simulink model "RRR_Robot_Control"  (R2021a)
settings: Solver=FixedStepAuto  StartTime=0.0  StopTime=10.0  FixedStep=0.001  RelTol=1e-3
values from neighbouring files (symbols this model uses):
  a = M\b    [parameters_Values.m]
  g = 9.81    [parameters_Values.m]
  L = [0.1,0.4,0.3]    [parameters_Values.m]
  m = [0.1,0.3,0.2]    [parameters_Values.m]
  r1 = 0.025    [parameters_Values.m]
libraries: pid_lib x3
settings Model: Creator=power  LastModifiedBy=power

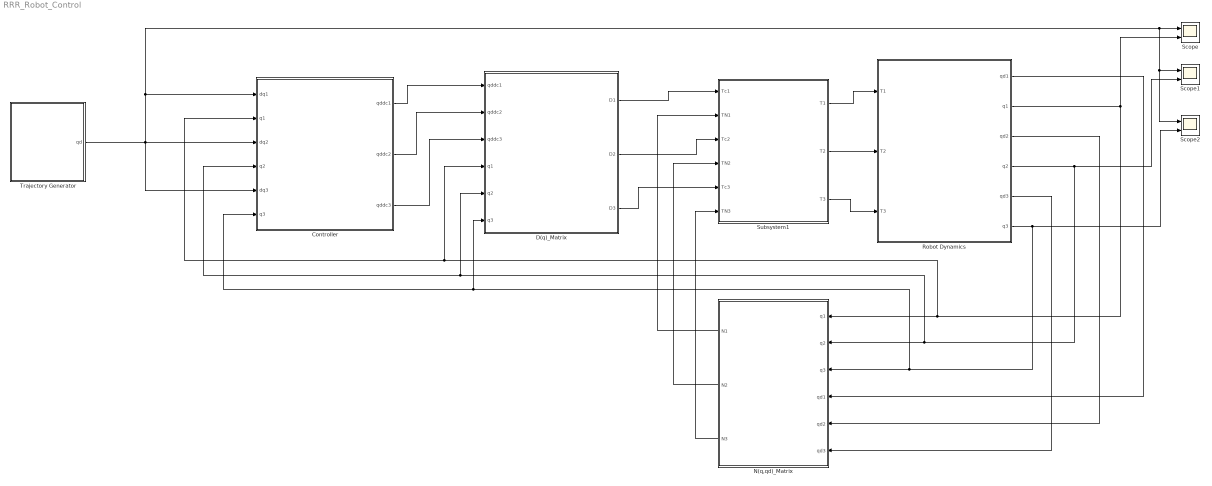
== system RRR_Robot_Control ==
  Controller : Subsystem
  D(q)_Matrix : Subsystem
  N(q,qd)_Matrix : Subsystem
  Robot Dynamics : Subsystem
  Scope : Scope  NumInputPorts=2
  Scope1 : Scope  NumInputPorts=2
  Scope2 : Scope  NumInputPorts=2
  Subsystem1 : Subsystem
  Trajectory Generator : Subsystem
  wires:
  Subsystem1/2(T2) -> Robot Dynamics/2(T2)
  Subsystem1/1(T1) -> Robot Dynamics/1(T1)
  Subsystem1/3(T3) -> Robot Dynamics/3(T3)
  N(q,qd)_Matrix/1(N1) -> Subsystem1/2(TN1)
  N(q,qd)_Matrix/2(N2) -> Subsystem1/4(TN2)
  N(q,qd)_Matrix/3(N3) -> Subsystem1/6(TN3)
  D(q)_Matrix/1(D1) -> Subsystem1/1(Tc1)
  D(q)_Matrix/2(D2) -> Subsystem1/3(Tc2)
  D(q)_Matrix/3(D3) -> Subsystem1/5(Tc3)
  Robot Dynamics/2(q1) -> Scope/2, Controller/2(q1), D(q)_Matrix/4(q1), N(q,qd)_Matrix/1(q1)
  Robot Dynamics/6(q3) -> Scope2/2, Controller/6(q3), D(q)_Matrix/6(q3), N(q,qd)_Matrix/3(q3)
  Robot Dynamics/4(q2) -> Scope1/2, Controller/4(q2), D(q)_Matrix/5(q2), N(q,qd)_Matrix/2(q2)
  Robot Dynamics/1(qd1) -> N(q,qd)_Matrix/4(qd1)
  Robot Dynamics/3(qd2) -> N(q,qd)_Matrix/5(qd2)
  Robot Dynamics/5(qd3) -> N(q,qd)_Matrix/6(qd3)
  Controller/1(qddc1) -> D(q)_Matrix/1(qddc1)
  Controller/2(qddc2) -> D(q)_Matrix/2(qddc2)
  Controller/3(qddc3) -> D(q)_Matrix/3(qddc3)
  Trajectory Generator/1(qd) -> Controller/5(dq3), Controller/3(dq2), Scope2/1, Scope1/1, Scope/1, Controller/1(dq1)

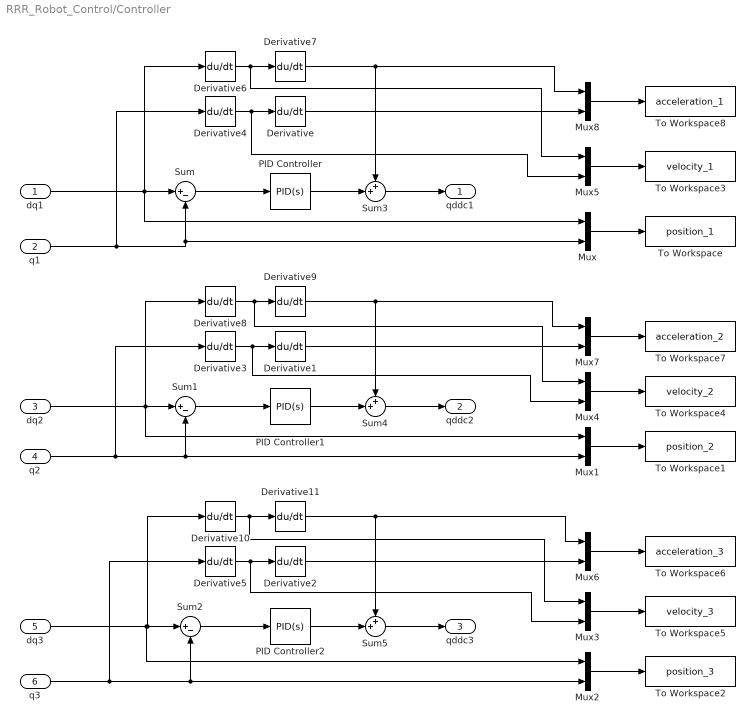
== system RRR_Robot_Control/Controller ==
  dq1 : Inport
  q1 : Inport  Port=2
  dq2 : Inport  Port=3
  q2 : Inport  Port=4
  dq3 : Inport  Port=5
  q3 : Inport  Port=6
  Derivative{,1..11} (12 alike) : Derivative
  Mux{,1..8} (9 alike) : Mux  Inputs=2
  PID Controller : pid_lib/PID Controller  Controller=PID  Form=Parallel  TimeDomain=Continuous-time  UseExternalTs=off  SampleTime=-1  IntegratorMethod=Forward Euler  FilterMethod=Forward Euler  ControllerParametersSource=internal  P=1  I=1  D=1  UseFilter=on  N=100  TunerSelectOption=Transfer Function Based (PID Tuner App)  InitialConditionSource=internal  InitialConditionForIntegrator=0  InitialConditionForFilter=0  DifferentiatorICPrevScaledInput=0  ExternalReset=none  TrackingMode=off  Kt=1  LimitOutput=off  SatLimitsSource=internal  UpperSaturationLimit=inf  LowerSaturationLimit=-inf  LinearizeAsGain=on  AntiWindupMode=none  Kb=1  POutMin=[]  POutMax=[]  IOutMin=[]  IOutMax=[]  DOutMin=[]  DOutMax=[]  NOutMin=[]  NOutMax=[]  SumOutMin=[]  SumOutMax=[]  SaturationOutMin=[]  SaturationOutMax=[]  PParamMin=[]  PParamMax=[]  IParamMin=[]  IParamMax=[]  DParamMin=[]  DParamMax=[]  NParamMin=[]  NParamMax=[]  KbParamMin=[]  KbParamMax=[]  KtParamMin=[]  KtParamMax=[]  KbOutMin=[]  KbOutMax=[]  KtOutMin=[]  KtOutMax=[]  IntegratorOutMin=[]  IntegratorOutMax=[]  FilterOutMin=[]  FilterOutMax=[]  SumI1OutMin=[]  SumI1OutMax=[]  SumI2OutMin=[]  SumI2OutMax=[]  SumI3OutMin=[]  SumI3OutMax=[]  SumI4OutMin=[]  SumI4OutMax=[]  SumDOutMin=[]  SumDOutMax=[]  DifferentiatorOutMin=[]  DifferentiatorOutMax=[]  FilterDiffOutCoefMin=[]  FilterDiffOutCoefMax=[]  ReciprocalOutMin=[]  ReciprocalOutMax=[]  SumDenOutMin=[]  SumDenOutMax=[]  SumNumOutMin=[]  SumNumOutMax=[]  DivideOutMin=[]  DivideOutMax=[]  UdiffTsProdOutMin=[]  UdiffTsProdOutMax=[]  NTsProdOutMin=[]  NTsProdOutMax=[]  UintegralTsProdOutMin=[]  UintegralTsProdOutMax=[]  UngainTsProdOutMin=[]  UngainTsProdOutMax=[]  IntegratorContinuousStateAttributes=''  IntegratorStateMustResolveToSignalObject=off  IntegratorRTWStateStorageClass=Auto  FilterContinuousStateAttributes=''  FilterStateMustResolveToSignalObject=off  FilterRTWStateStorageClass=Auto  ParallelPVariant=InternalParameters  IdealPVariant=Disabled  IVariant=InternalParameters  DVariant=InternalParameters  IntegratorVariant=Continuous  SatVariant=Disabled  AWVariant=Passthrough  PCopyVariant=Disabled  TRVariant=Disabled  FdbkBlocksVariant=Forward  IdealPFdbkVariant=Disabled  SatFdbkVariant=Disabled  DerivativeFilterVariant=ContFilter  NVariant=InternalParameters  NCopyVariant=Disabled  FilterICVariant=InternalICsFilter  IntegratorICVariant=InternalICs  ExternalResetVariant=Disabled  TRSumVariant=Passthrough  SumFdbkVariant=Disabled  SumVariant=Sum_PID  TsampFilterVariant=InternalTs  TsampNgainVariant=Passthrough  TsampIntegralVariant=Passthrough  ExternalSaturationOutDataTypeStr=Inherit: Same as second input
  PID Controller1 : pid_lib/PID Controller  Controller=PID  Form=Parallel  TimeDomain=Continuous-time  UseExternalTs=off  SampleTime=-1  IntegratorMethod=Forward Euler  FilterMethod=Forward Euler  ControllerParametersSource=internal  P=1  I=1  D=1  UseFilter=on  N=100  TunerSelectOption=Transfer Function Based (PID Tuner App)  InitialConditionSource=internal  InitialConditionForIntegrator=0  InitialConditionForFilter=0  DifferentiatorICPrevScaledInput=0  ExternalReset=none  TrackingMode=off  Kt=1  LimitOutput=off  SatLimitsSource=internal  UpperSaturationLimit=inf  LowerSaturationLimit=-inf  LinearizeAsGain=on  AntiWindupMode=none  Kb=1  POutMin=[]  POutMax=[]  IOutMin=[]  IOutMax=[]  DOutMin=[]  DOutMax=[]  NOutMin=[]  NOutMax=[]  SumOutMin=[]  SumOutMax=[]  SaturationOutMin=[]  SaturationOutMax=[]  PParamMin=[]  PParamMax=[]  IParamMin=[]  IParamMax=[]  DParamMin=[]  DParamMax=[]  NParamMin=[]  NParamMax=[]  KbParamMin=[]  KbParamMax=[]  KtParamMin=[]  KtParamMax=[]  KbOutMin=[]  KbOutMax=[]  KtOutMin=[]  KtOutMax=[]  IntegratorOutMin=[]  IntegratorOutMax=[]  FilterOutMin=[]  FilterOutMax=[]  SumI1OutMin=[]  SumI1OutMax=[]  SumI2OutMin=[]  SumI2OutMax=[]  SumI3OutMin=[]  SumI3OutMax=[]  SumI4OutMin=[]  SumI4OutMax=[]  SumDOutMin=[]  SumDOutMax=[]  DifferentiatorOutMin=[]  DifferentiatorOutMax=[]  FilterDiffOutCoefMin=[]  FilterDiffOutCoefMax=[]  ReciprocalOutMin=[]  ReciprocalOutMax=[]  SumDenOutMin=[]  SumDenOutMax=[]  SumNumOutMin=[]  SumNumOutMax=[]  DivideOutMin=[]  DivideOutMax=[]  UdiffTsProdOutMin=[]  UdiffTsProdOutMax=[]  NTsProdOutMin=[]  NTsProdOutMax=[]  UintegralTsProdOutMin=[]  UintegralTsProdOutMax=[]  UngainTsProdOutMin=[]  UngainTsProdOutMax=[]  IntegratorContinuousStateAttributes=''  IntegratorStateMustResolveToSignalObject=off  IntegratorRTWStateStorageClass=Auto  FilterContinuousStateAttributes=''  FilterStateMustResolveToSignalObject=off  FilterRTWStateStorageClass=Auto  ParallelPVariant=InternalParameters  IdealPVariant=Disabled  IVariant=InternalParameters  DVariant=InternalParameters  IntegratorVariant=Continuous  SatVariant=Disabled  AWVariant=Passthrough  PCopyVariant=Disabled  TRVariant=Disabled  FdbkBlocksVariant=Forward  IdealPFdbkVariant=Disabled  SatFdbkVariant=Disabled  DerivativeFilterVariant=ContFilter  NVariant=InternalParameters  NCopyVariant=Disabled  FilterICVariant=InternalICsFilter  IntegratorICVariant=InternalICs  ExternalResetVariant=Disabled  TRSumVariant=Passthrough  SumFdbkVariant=Disabled  SumVariant=Sum_PID  TsampFilterVariant=InternalTs  TsampNgainVariant=Passthrough  TsampIntegralVariant=Passthrough  ExternalSaturationOutDataTypeStr=Inherit: Same as second input
  PID Controller2 : pid_lib/PID Controller  Controller=PID  Form=Parallel  TimeDomain=Continuous-time  UseExternalTs=off  SampleTime=-1  IntegratorMethod=Forward Euler  FilterMethod=Forward Euler  ControllerParametersSource=internal  P=1  I=1  D=1  UseFilter=on  N=100  TunerSelectOption=Transfer Function Based (PID Tuner App)  InitialConditionSource=internal  InitialConditionForIntegrator=0  InitialConditionForFilter=0  DifferentiatorICPrevScaledInput=0  ExternalReset=none  TrackingMode=off  Kt=1  LimitOutput=off  SatLimitsSource=internal  UpperSaturationLimit=inf  LowerSaturationLimit=-inf  LinearizeAsGain=on  AntiWindupMode=none  Kb=1  POutMin=[]  POutMax=[]  IOutMin=[]  IOutMax=[]  DOutMin=[]  DOutMax=[]  NOutMin=[]  NOutMax=[]  SumOutMin=[]  SumOutMax=[]  SaturationOutMin=[]  SaturationOutMax=[]  PParamMin=[]  PParamMax=[]  IParamMin=[]  IParamMax=[]  DParamMin=[]  DParamMax=[]  NParamMin=[]  NParamMax=[]  KbParamMin=[]  KbParamMax=[]  KtParamMin=[]  KtParamMax=[]  KbOutMin=[]  KbOutMax=[]  KtOutMin=[]  KtOutMax=[]  IntegratorOutMin=[]  IntegratorOutMax=[]  FilterOutMin=[]  FilterOutMax=[]  SumI1OutMin=[]  SumI1OutMax=[]  SumI2OutMin=[]  SumI2OutMax=[]  SumI3OutMin=[]  SumI3OutMax=[]  SumI4OutMin=[]  SumI4OutMax=[]  SumDOutMin=[]  SumDOutMax=[]  DifferentiatorOutMin=[]  DifferentiatorOutMax=[]  FilterDiffOutCoefMin=[]  FilterDiffOutCoefMax=[]  ReciprocalOutMin=[]  ReciprocalOutMax=[]  SumDenOutMin=[]  SumDenOutMax=[]  SumNumOutMin=[]  SumNumOutMax=[]  DivideOutMin=[]  DivideOutMax=[]  UdiffTsProdOutMin=[]  UdiffTsProdOutMax=[]  NTsProdOutMin=[]  NTsProdOutMax=[]  UintegralTsProdOutMin=[]  UintegralTsProdOutMax=[]  UngainTsProdOutMin=[]  UngainTsProdOutMax=[]  IntegratorContinuousStateAttributes=''  IntegratorStateMustResolveToSignalObject=off  IntegratorRTWStateStorageClass=Auto  FilterContinuousStateAttributes=''  FilterStateMustResolveToSignalObject=off  FilterRTWStateStorageClass=Auto  ParallelPVariant=InternalParameters  IdealPVariant=Disabled  IVariant=InternalParameters  DVariant=InternalParameters  IntegratorVariant=Continuous  SatVariant=Disabled  AWVariant=Passthrough  PCopyVariant=Disabled  TRVariant=Disabled  FdbkBlocksVariant=Forward  IdealPFdbkVariant=Disabled  SatFdbkVariant=Disabled  DerivativeFilterVariant=ContFilter  NVariant=InternalParameters  NCopyVariant=Disabled  FilterICVariant=InternalICsFilter  IntegratorICVariant=InternalICs  ExternalResetVariant=Disabled  TRSumVariant=Passthrough  SumFdbkVariant=Disabled  SumVariant=Sum_PID  TsampFilterVariant=InternalTs  TsampNgainVariant=Passthrough  TsampIntegralVariant=Passthrough  ExternalSaturationOutDataTypeStr=Inherit: Same as second input
  Sum : Sum  Inputs=|+-
  Sum1 : Sum  Inputs=|+-
  Sum2 : Sum  Inputs=|+-
  Sum3 : Sum  Inputs=++|
  Sum4 : Sum  Inputs=++|
  Sum5 : Sum  Inputs=++|
  To Workspace : ToWorkspace  VariableName=position_1  SaveFormat=Timeseries  SampleTime=0.05
  To Workspace1 : ToWorkspace  VariableName=position_2  SaveFormat=Timeseries  SampleTime=0.05
  To Workspace2 : ToWorkspace  VariableName=position_3  SaveFormat=Timeseries  SampleTime=0.05
  To Workspace3 : ToWorkspace  VariableName=velocity_1  SaveFormat=Timeseries  SampleTime=0.05
  To Workspace4 : ToWorkspace  VariableName=velocity_2  SaveFormat=Timeseries  SampleTime=0.05
  To Workspace5 : ToWorkspace  VariableName=velocity_3  SaveFormat=Timeseries  SampleTime=0.05
  To Workspace6 : ToWorkspace  VariableName=acceleration_3  SaveFormat=Timeseries  SampleTime=0.05
  To Workspace7 : ToWorkspace  VariableName=acceleration_2  SaveFormat=Timeseries  SampleTime=0.05
  To Workspace8 : ToWorkspace  VariableName=acceleration_1  SaveFormat=Timeseries  SampleTime=0.05
  qddc1 : Outport
  qddc2 : Outport  Port=2
  qddc3 : Outport  Port=3
  wires:
  Sum/1 -> PID Controller/1
  Sum1/1 -> PID Controller1/1
  Sum2/1 -> PID Controller2/1
  dq1/1 -> Derivative6/1, Mux/1, Sum/1
  q1/1 -> Derivative4/1, Sum/2, Mux/2
  dq2/1 -> Derivative8/1, Mux1/1, Sum1/1
  q2/1 -> Derivative3/1, Mux1/2, Sum1/2
  dq3/1 -> Mux2/1, Derivative10/1, Sum2/1
  q3/1 -> Derivative5/1, Sum2/2, Mux2/2
  PID Controller2/1 -> Sum5/2
  Sum5/1 -> qddc3/1
  Derivative2/1 -> Mux6/2
  Sum4/1 -> qddc2/1
  PID Controller1/1 -> Sum4/2
  Sum3/1 -> qddc1/1
  PID Controller/1 -> Sum3/2
  Derivative3/1 -> Mux4/2, Derivative1/1
  Derivative4/1 -> Mux5/2, Derivative/1
  Derivative5/1 -> Mux3/2, Derivative2/1
  Derivative/1 -> Mux8/2
  Derivative1/1 -> Mux7/2
  Mux/1 -> To Workspace/1
  Mux1/1 -> To Workspace1/1
  Mux2/1 -> To Workspace2/1
  Mux3/1 -> To Workspace5/1
  Mux4/1 -> To Workspace4/1
  Mux5/1 -> To Workspace3/1
  Derivative6/1 -> Mux5/1, Derivative7/1
  Derivative8/1 -> Mux4/1, Derivative9/1
  Derivative10/1 -> Mux3/1, Derivative11/1
  Mux6/1 -> To Workspace6/1
  Derivative11/1 -> Sum5/1, Mux6/1
  Mux7/1 -> To Workspace7/1
  Derivative9/1 -> Sum4/1, Mux7/1
  Mux8/1 -> To Workspace8/1
  Derivative7/1 -> Sum3/1, Mux8/1

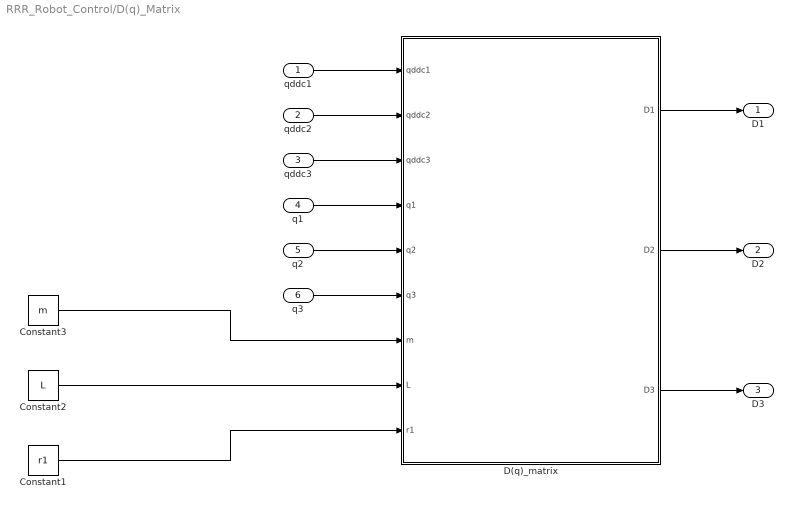
== system RRR_Robot_Control/D(q)_Matrix ==
  qddc1 : Inport
  qddc2 : Inport  Port=2
  qddc3 : Inport  Port=3
  q1 : Inport  Port=4
  q2 : Inport  Port=5
  q3 : Inport  Port=6
  Constant1 : Constant  Value=r1
  Constant2 : Constant  Value=L
  Constant3 : Constant  Value=m
  D(q)_matrix : MATLAB Function  TreatAsAtomicUnit=on
  D1 : Outport
  D2 : Outport  Port=2
  D3 : Outport  Port=3
  wires:
  D(q)_matrix/1(D1) -> D1/1
  D(q)_matrix/2(D2) -> D2/1
  D(q)_matrix/3(D3) -> D3/1
  qddc1/1 -> D(q)_matrix/1(qddc1)
  qddc2/1 -> D(q)_matrix/2(qddc2)
  qddc3/1 -> D(q)_matrix/3(qddc3)
  Constant1/1 -> D(q)_matrix/9(r1)
  Constant2/1 -> D(q)_matrix/8(L)
  Constant3/1 -> D(q)_matrix/7(m)
  q1/1 -> D(q)_matrix/4(q1)
  q2/1 -> D(q)_matrix/5(q2)
  q3/1 -> D(q)_matrix/6(q3)

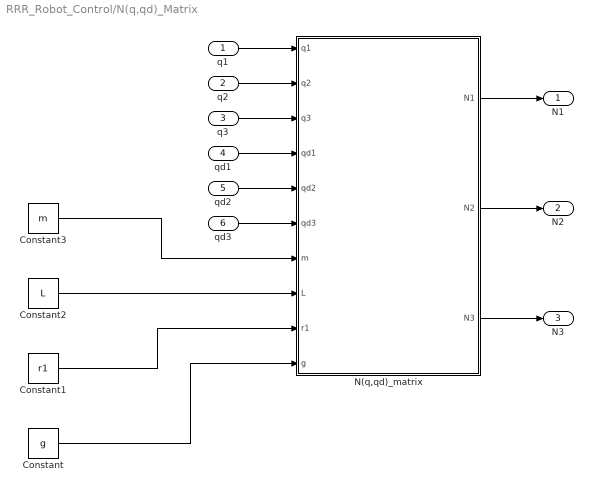
== system RRR_Robot_Control/N(q,qd)_Matrix ==
  q1 : Inport
  q2 : Inport  Port=2
  q3 : Inport  Port=3
  qd1 : Inport  Port=4
  qd2 : Inport  Port=5
  qd3 : Inport  Port=6
  Constant : Constant  Value=g
  Constant1 : Constant  Value=r1
  Constant2 : Constant  Value=L
  Constant3 : Constant  Value=m
  N(q,qd)_matrix : MATLAB Function  TreatAsAtomicUnit=on
  N1 : Outport
  N2 : Outport  Port=2
  N3 : Outport  Port=3
  wires:
  q1/1 -> N(q,qd)_matrix/1(q1)
  N(q,qd)_matrix/1(N1) -> N1/1
  N(q,qd)_matrix/2(N2) -> N2/1
  N(q,qd)_matrix/3(N3) -> N3/1
  q2/1 -> N(q,qd)_matrix/2(q2)
  q3/1 -> N(q,qd)_matrix/3(q3)
  qd2/1 -> N(q,qd)_matrix/5(qd2)
  qd1/1 -> N(q,qd)_matrix/4(qd1)
  qd3/1 -> N(q,qd)_matrix/6(qd3)
  Constant/1 -> N(q,qd)_matrix/10(g)
  Constant1/1 -> N(q,qd)_matrix/9(r1)
  Constant2/1 -> N(q,qd)_matrix/8(L)
  Constant3/1 -> N(q,qd)_matrix/7(m)

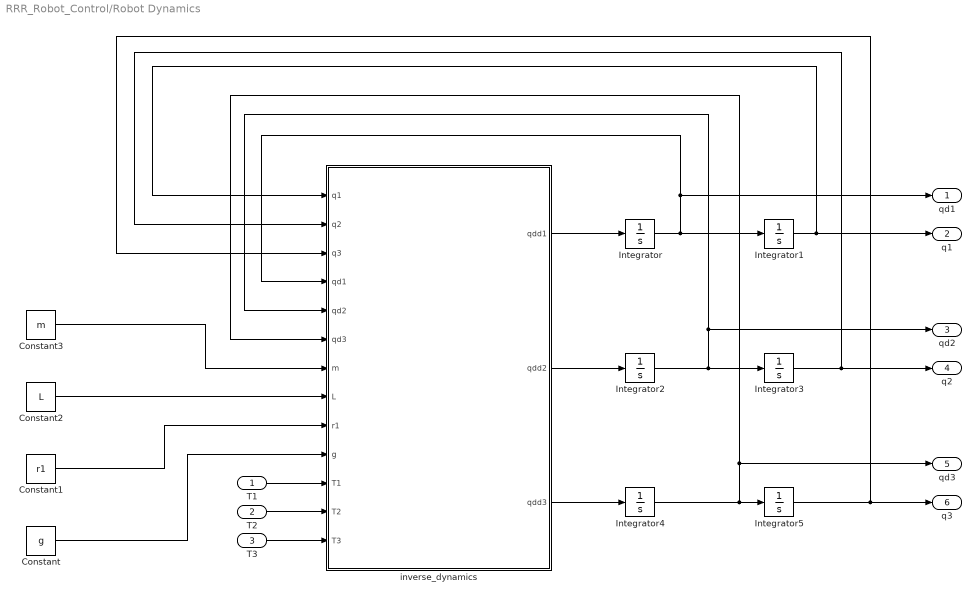
== system RRR_Robot_Control/Robot Dynamics ==
  T1 : Inport
  T2 : Inport  Port=2
  T3 : Inport  Port=3
  Constant : Constant  Value=g
  Constant1 : Constant  Value=r1
  Constant2 : Constant  Value=L
  Constant3 : Constant  Value=m
  Integrator{,1..5} (6 alike) : Integrator
  inverse_dynamics : MATLAB Function  TreatAsAtomicUnit=on
  qd1 : Outport
  q1 : Outport  Port=2
  qd2 : Outport  Port=3
  q2 : Outport  Port=4
  qd3 : Outport  Port=5
  q3 : Outport  Port=6
  wires:
  T1/1 -> inverse_dynamics/11(T1)
  inverse_dynamics/1(qdd1) -> Integrator/1
  Integrator/1 -> qd1/1, inverse_dynamics/4(qd1), Integrator1/1
  Integrator1/1 -> q1/1, inverse_dynamics/1(q1)
  inverse_dynamics/2(qdd2) -> Integrator2/1
  Integrator2/1 -> qd2/1, inverse_dynamics/5(qd2), Integrator3/1
  inverse_dynamics/3(qdd3) -> Integrator4/1
  Integrator4/1 -> qd3/1, inverse_dynamics/6(qd3), Integrator5/1
  Integrator5/1 -> q3/1, inverse_dynamics/3(q3)
  Constant/1 -> inverse_dynamics/10(g)
  Constant1/1 -> inverse_dynamics/9(r1)
  Constant2/1 -> inverse_dynamics/8(L)
  Constant3/1 -> inverse_dynamics/7(m)
  Integrator3/1 -> inverse_dynamics/2(q2), q2/1
  T2/1 -> inverse_dynamics/12(T2)
  T3/1 -> inverse_dynamics/13(T3)

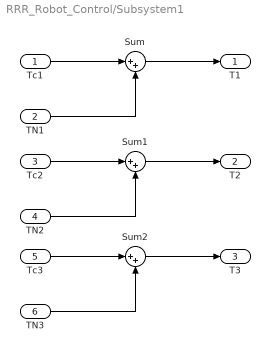
== system RRR_Robot_Control/Subsystem1 ==
  Tc1 : Inport
  TN1 : Inport  Port=2
  Tc2 : Inport  Port=3
  TN2 : Inport  Port=4
  Tc3 : Inport  Port=5
  TN3 : Inport  Port=6
  Sum : Sum  Inputs=|++
  Sum1 : Sum  Inputs=|++
  Sum2 : Sum  Inputs=|++
  T1 : Outport
  T2 : Outport  Port=2
  T3 : Outport  Port=3
  wires:
  Sum/1 -> T1/1
  Tc1/1 -> Sum/1
  TN1/1 -> Sum/2
  TN2/1 -> Sum1/2
  Tc2/1 -> Sum1/1
  Sum1/1 -> T2/1
  Sum2/1 -> T3/1
  Tc3/1 -> Sum2/1
  TN3/1 -> Sum2/2

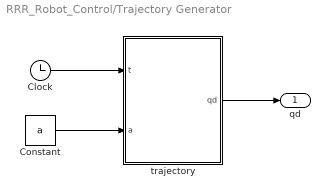
== system RRR_Robot_Control/Trajectory Generator ==
  Clock : Clock
  Constant : Constant  Value=a
  trajectory : MATLAB Function  TreatAsAtomicUnit=on
  qd : Outport
  wires:
  trajectory/1(qd) -> qd/1
  Clock/1 -> trajectory/1(t)
  Constant/1 -> trajectory/2(a)

== matlab function RRR_Robot_Control/Robot Dynamics/inverse_dynamics ==
  data: q1 input; q2 input; q3 input; qdd1 output; qd1 input; qd2 input; qd3 input; m input; L input; r1 input; g input; T1 input; qdd2 output; qdd3 output; T2 input; T3 input
function [qdd1,qdd2,qdd3] = inverse_dynamics(q1, q2, q3, qd1, qd2, qd3, m, L, r1, g, T1, T2, T3)
    %Parameters
    m1 = m(1); m2 = m(2); m3 = m(3);
    L1 = L(1); L2 = L(2); L3 = L(3);
    %Output
    qdd1 = (6*T1 + 2*L2^2*m2*qd1*qd2*sin(2*q2) + 6*L2^2*m3*qd1*qd2*sin(2*q2) + 2*L3^2*m3*qd1*qd2*sin(2*q2 + 2*q3) + 2*L3^2*m3*qd1*qd3*sin(2*q2 + 2*q3) + 3*L2*L3*m3*qd1*qd3*sin(q3) + 6*L2*L3*m3*qd1*qd2*sin(2*q2 + q3) + 3*L2*L3*m3*qd1*qd3*sin(2*q2 + q3))/(L2^2*m2 + 3*L2^2*m3 + L3^2*m3 + 3*m1*r1^2 + L2^2*m2*cos(2*q2) + 3*L2^2*m3*cos(2*q2) + L3^2*m3*cos(2*q2 + 2*q3) + 3*L2*L3*m3*cos(q3) + 3*L2*L3*m3*cos(2*q2 + q3));
    qdd2 = (48*L3*T2 - 48*L3*T3 - 72*L2*T3*cos(q3) + 9*L2^2*L3*m3*qd1^2*sin(2*q2 + 2*q3) + 6*L2*L3^2*m3*qd1^2*sin(2*q2 + 3*q3) + 12*L2*L3^2*m3*qd1^2*sin(q3) + 24*L2*L3^2*m3*qd2^2*sin(q3) + 24*L2*L3^2*m3*qd3^2*sin(q3) - 24*L2*L3*g*m2*cos(q2) - 30*L2*L3*g*m3*cos(q2) - 6*L2*L3^2*m3*qd1^2*sin(2*q2 + q3) + 18*L2*L3*g*m3*cos(q2 + 2*q3) - 8*L2^2*L3*m2*qd1^2*sin(2*q2) - 15*L2^2*L3*m3*qd1^2*sin(2*q2) + 9*L2^2*L3*m3*qd1^2*sin(2*q3) + 18*L2^2*L3*m3*qd2^2*sin(2*q3) + 48*L2*L3^2*m3*qd2*qd3*sin(q3))/(2*L2^2*L3*(8*m2 + 15*m3 - 9*m3*cos(2*q3)));
    qdd3 = -(24*L3^2*T2*m3 - 72*L2^2*T3*m3 - 24*L2^2*T3*m2 - 24*L3^2*T3*m3 - 3*L2*L3^3*m3^2*qd1^2*sin(2*q2 + q3) + 9*L2^3*L3*m3^2*qd1^2*sin(2*q2 + q3) + 18*L2^2*L3*g*m3^2*cos(q2 + q3) - 15*L2*L3^2*g*m3^2*cos(q2) - 9*L2^3*L3*m3^2*qd1^2*sin(2*q2 - q3) + 3*L2*L3^3*m3^2*qd1^2*sin(2*q2 + 3*q3) + 36*L2*L3*T2*m3*cos(q3) - 72*L2*L3*T3*m3*cos(q3) - 18*L2^2*L3*g*m3^2*cos(q2 - q3) + 9*L2*L3^2*g*m3^2*cos(q2 + 2*q3) - 12*L2^2*L3^2*m3^2*qd1^2*sin(2*q2) + 9*L2^2*L3^2*m3^2*qd1^2*sin(2*q3) + 18*L2^2*L3^2*m3^2*qd2^2*sin(2*q3) + 9*L2^2*L3^2*m3^2*qd3^2*sin(2*q3) + 12*L2^2*L3^2*m3^2*qd1^2*sin(2*q2 + 2*q3) + 6*L2*L3^3*m3^2*qd1^2*sin(q3) + 18*L2^3*L3*m3^2*qd1^2*sin(q3) + 12*L2*L3^3*m3^2*qd2^2*sin(q3) + 36*L2^3*L3*m3^2*qd2^2*sin(q3) + 12*L2*L3^3*m3^2*qd3^2*sin(q3) + 3*L2^3*L3*m2*m3*qd1^2*sin(2*q2 + q3) + 3*L2^2*L3*g*m2*m3*cos(q2 + q3) - 12*L2*L3^2*g*m2*m3*cos(q2) - 3*L2^3*L3*m2*m3*qd1^2*sin(2*q2 - q3) - 9*L2^2*L3*g*m2*m3*cos(q2 - q3) - 4*L2^2*L3^2*m2*m3*qd1^2*sin(2*q2) + 18*L2^2*L3^2*m3^2*qd2*qd3*sin(2*q3) + 4*L2^2*L3^2*m2*m3*qd1^2*sin(2*q2 + 2*q3) + 6*L2^3*L3*m2*m3*qd1^2*sin(q3) + 12*L2^3*L3*m2*m3*qd2^2*sin(q3) + 24*L2*L3^3*m3^2*qd2*qd3*sin(q3))/(L2^2*L3^2*m3*(8*m2 + 15*m3 - 9*m3*cos(2*q3)));
    
end

== matlab function RRR_Robot_Control/D(q)_Matrix/D(q)_matrix ==
  data: qddc1 input; D1 output; qddc2 input; qddc3 input; q1 input; q2 input; q3 input; m input; L input; r1 input; D2 output; D3 output
function [D1,D2,D3] = D_matrix(qddc1, qddc2, qddc3, q1, q2, q3, m, L, r1)
    %Parameters
    m1 = m(1); m2 = m(2); m3 = m(3);
    L1 = L(1); L2 = L(2); L3 = L(3);
    %Equations
    D = [(L2^2*m2)/6 + (L2^2*m3)/2 + (L3^2*m3)/6 + (m1*r1^2)/2 + (L2^2*m2*cos(2*q2))/6 + (L2^2*m3*cos(2*q2))/2 + (L3^2*m3*cos(2*q2 + 2*q3))/6 + (L2*L3*m3*cos(q3))/2 + (L2*L3*m3*cos(2*q2 + q3))/2, 0, 0;
        0, (L2^2*m2)/3 + L2^2*m3 + (L3^2*m3)/3 + L2*L3*m3*cos(q3), (L3*m3*(2*L3 + 3*L2*cos(q3)))/6;
        0, (L3*m3*(2*L3 + 3*L2*cos(q3)))/6, (L3^2*m3)/3];
    Dc = D*[qddc1;qddc2;qddc3];
    %Output
    D1 = Dc(1); D2 = Dc(2); D3 = Dc(3);
end

== matlab function RRR_Robot_Control/N(q,qd)_Matrix/N(q,qd)_matrix ==
  data: q1 input; N1 output; q2 input; q3 input; qd1 input; qd2 input; qd3 input; m input; L input; r1 input; g input; N2 output; N3 output
function [N1,N2,N3] = N_matrix(q1, q2, q3, qd1, qd2, qd3, m, L, r1, g)
    %Parameters
    m1 = m(1); m2 = m(2); m3 = m(3);
    L1 = L(1); L2 = L(2); L3 = L(3);
    %Equations
    N = [- qd1*qd2*((L2^2*m2*sin(2*q2))/3 + L2^2*m3*sin(2*q2) + (L3^2*m3*sin(2*q2 + 2*q3))/3 + L2*L3*m3*sin(2*q2 + q3)) - (L3*m3*qd1*qd3*(2*L3*sin(2*q2 + 2*q3) + 3*L2*sin(q3) + 3*L2*sin(2*q2 + q3)))/6;
        ((L2^2*m2*sin(2*q2))/6 + (L2^2*m3*sin(2*q2))/2 + (L3^2*m3*sin(2*q2 + 2*q3))/6 + (L2*L3*m3*sin(2*q2 + q3))/2)*qd1^2 + g*m3*((L3*cos(q2 + q3))/2 + L2*cos(q2)) + (L2*g*m2*cos(q2))/2 - (L2*L3*m3*qd3^2*sin(q3))/2 - L2*L3*m3*qd2*qd3*sin(q3);
        (L3*m3*(6*g*cos(q2 + q3) + 3*L2*qd1^2*sin(q3) + 6*L2*qd2^2*sin(q3) + 3*L2*qd1^2*sin(2*q2 + q3) + 2*L3*qd1^2*sin(2*q2 + 2*q3)))/12];
    %Output
    N1 = N(1); N2 = N(2); N3 = N(3);
end

== matlab function RRR_Robot_Control/Trajectory Generator/trajectory ==
  data: t input; qd output; a input
function qd = trajectory(t, a)
    qd = a(1) + a(2)*t +a(3)*t^2 + a(4)*t^3 +a(5)*t^4 + a(6)*t^5;
end
